simulink model "model12"  (R2013a)
settings: Solver=ode45  StartTime=0.0  StopTime=10.0  RelTol=1e-3
settings Model: Creator=Axel  LastModifiedBy=Axel
settings OptimizationCC: InlineParams=on

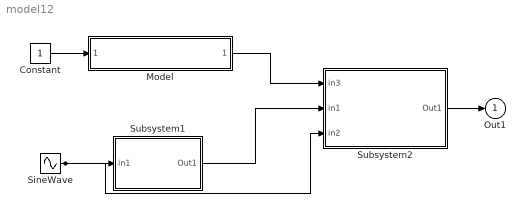
== system model12 ==
  Constant : Constant
  Model : ModelReference  ModelNameDialog=model3  ModelReferenceVersion=1.4  CopyOfModelName=model3  DefaultDataLogging=on
  SineWave : Sin
  Subsystem1 : Subsystem
  Subsystem2 : Subsystem
  Out1 : Outport
  wires:
  Subsystem2/1(Out1) -> Out1/1
  Subsystem1/1(Out1) -> Subsystem2/2(in1)
  Constant/1 -> Model/1
  SineWave/1 -> Subsystem2/3(in2), Subsystem1/1(in1)
  Model/1 -> Subsystem2/1(in3)

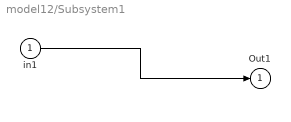
== system model12/Subsystem1 ==
  in1 : Inport
  Out1 : Outport
  wires:
  in1/1 -> Out1/1

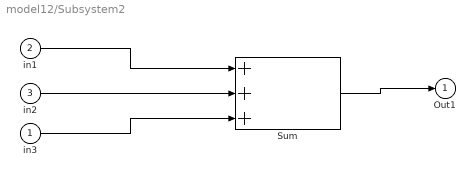
== system model12/Subsystem2 ==
  in3 : Inport
  in1 : Inport  Port=2
  in2 : Inport  Port=3
  Sum : Sum  Inputs=|+++  SaturateOnIntegerOverflow=on  InputSameDT=on  OutDataTypeStr=Inherit: Same as first input
  Out1 : Outport
  wires:
  Sum/1 -> Out1/1
  in3/1 -> Sum/3
  in2/1 -> Sum/2
  in1/1 -> Sum/1
